simulink model "Respuesta_realDelSisistema_antecambios_en_entrada"  (R2019a)
settings: Solver=VariableStepAuto  StartTime=0.0  StopTime=9000  RelTol=1e-3
settings Model: Creator=Beto  LastModifiedBy=Beto

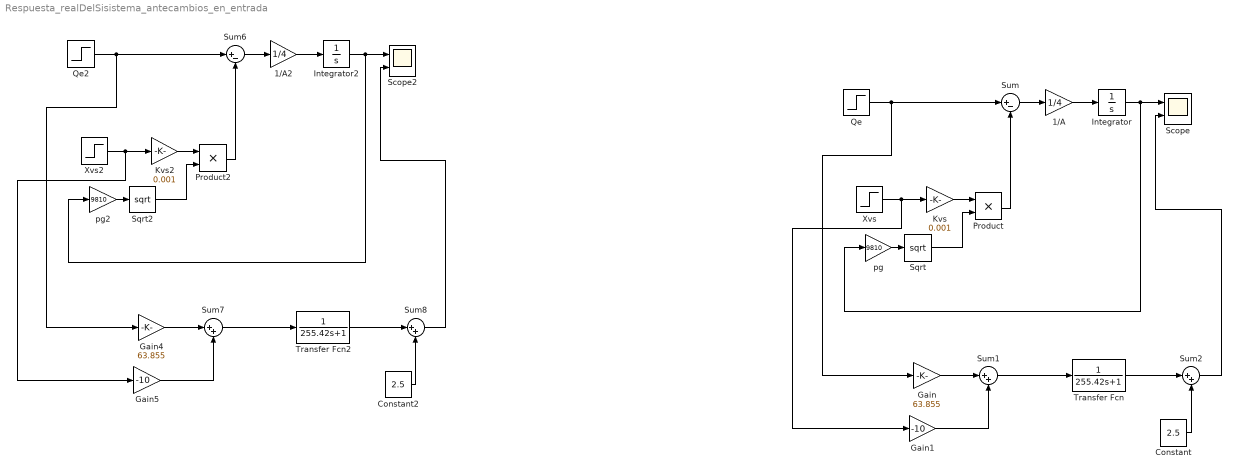
== system Respuesta_realDelSisistema_antecambios_en_entrada ==
  1/A : Gain  Gain=1/4
  1/A2 : Gain  Gain=1/4
  Constant : Constant  Value=2.5
  Constant2 : Constant  Value=2.5
  Gain : Gain  Gain=63.855
  Gain1 : Gain  Gain=-10
  Gain4 : Gain  Gain=63.855
  Gain5 : Gain  Gain=-10
  Integrator : Integrator
  Integrator2 : Integrator
  Kvs : Gain  Gain=0.001
  Kvs2 : Gain  Gain=0.001
  Product : Product
  Product2 : Product
  Qe : Step  Time=2000  Before=0.078  After=0.07722  SampleTime=0.1
  Qe2 : Step  Time=2000  Before=0.078  After=0.0702  SampleTime=0.1
  Scope : Scope  NumInputPorts=2
  Scope2 : Scope  NumInputPorts=2
  Sqrt : Sqrt  SaturateOnIntegerOverflow=on
  Sqrt2 : Sqrt  SaturateOnIntegerOverflow=on
  Sum : Sum  Inputs=|+-
  Sum{1..2,7..8} (4 alike) : Sum  Inputs=|++
  Sum6 : Sum  Inputs=|+-
  Transfer Fcn : TransferFcn  Denominator=[255.42 1]
  Transfer Fcn2 : TransferFcn  Denominator=[255.42 1]
  Xvs : Step  Time=4000  Before=0.5  After=0.49  SampleTime=0
  Xvs2 : Step  Time=4000  Before=0.5  After=0.4  SampleTime=0
  pg : Gain  Gain=9810
  pg2 : Gain  Gain=9810
  wires:
  Sum/1 -> 1/A/1
  1/A/1 -> Integrator/1
  Kvs/1 -> Product/1
  Integrator/1 -> Scope/1, pg/1
  pg/1 -> Sqrt/1
  Sqrt/1 -> Product/2
  Product/1 -> Sum/2
  Gain1/1 -> Sum1/2
  Gain/1 -> Sum1/1
  Sum1/1 -> Transfer Fcn/1
  Transfer Fcn/1 -> Sum2/1
  Qe/1 -> Gain/1, Sum/1
  Xvs/1 -> Gain1/1, Kvs/1
  Constant/1 -> Sum2/2
  Sum2/1 -> Scope/2
  Integrator2/1 -> Scope2/1, pg2/1
  Sqrt2/1 -> Product2/2
  Sum6/1 -> 1/A2/1
  Gain4/1 -> Sum7/1
  Kvs2/1 -> Product2/1
  1/A2/1 -> Integrator2/1
  pg2/1 -> Sqrt2/1
  Sum7/1 -> Transfer Fcn2/1
  Product2/1 -> Sum6/2
  Gain5/1 -> Sum7/2
  Xvs2/1 -> Gain5/1, Kvs2/1
  Qe2/1 -> Gain4/1, Sum6/1
  Constant2/1 -> Sum8/2
  Transfer Fcn2/1 -> Sum8/1
  Sum8/1 -> Scope2/2
